simulink model "ad3ab2"  (Simulink 4.00)
settings: Solver=ode45  SolverMode=SingleTasking  StartTime=0.0  StopTime=0.2  RelTol=1e-4  AbsTol=1e-8
CloseFcn:
  | ;slview('closediagram',bdroot);
settings Model: LimitDataPoints=off  BlockReductionOpt=off

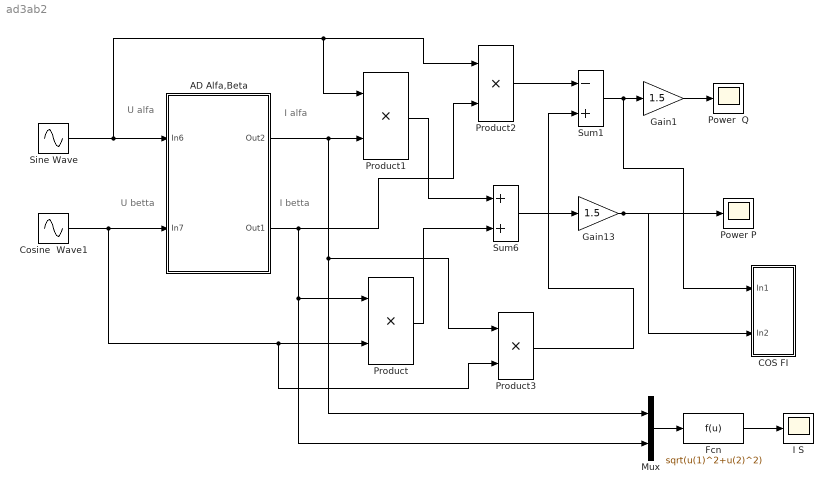
== system ad3ab2 ==
  note: I alfa
  note: I betta
  note: U alfa
  note: U betta
  AD Alfa,Beta : Subsystem
      settings: RTWFcnNameOpts=Auto  RTWFileNameOpts=Auto
  COS FI : Subsystem
      settings: RTWFcnNameOpts=Auto  RTWFileNameOpts=Auto
  Cosine  Wave1 : Sin  SineType=Time-based  Amplitude=311  Bias=0  Frequency=314  Phase=-pi/2  Samples=10  SampleTime=0  Offset=0
  Fcn : Fcn  Expr=sqrt(u(1)^2+u(2)^2)
  Gain1 : Gain  Gain=1.5  Multiplication=Element-wise(K.*u)  SaturateOnIntegerOverflow=on
  Gain13 : Gain  Gain=1.5  Multiplication=Element-wise(K.*u)  SaturateOnIntegerOverflow=on
  I S : Scope
      settings: TickLabels=on  TimeRange=80  YMin=-1  YMax=2  SaveToWorkspace=off  SaveName=ScopeData5  DataFormat=Array  MaxDataPoints=5000
  Mux : Mux  Inputs=2
  Power  Q : Scope
      settings: TickLabels=on  TimeRange=80  YMin=-1  YMax=2  SaveToWorkspace=off  SaveName=ScopeData3  DataFormat=Array  MaxDataPoints=5000
  Power P : Scope
      settings: TickLabels=on  TimeRange=80  YMin=-1  YMax=2  SaveToWorkspace=off  SaveName=ScopeData2  DataFormat=Array  MaxDataPoints=5000
  Product{,1..3} (4 alike) : Product  Inputs=2  Multiplication=Element-wise(.*)  SaturateOnIntegerOverflow=on
  Sine Wave : Sin  SineType=Time-based  Amplitude=311  Bias=0  Frequency=314  Phase=0  Samples=10  SampleTime=0  Offset=0
  Sum1 : Sum  Inputs=-+  SaturateOnIntegerOverflow=on
  Sum6 : Sum  Inputs=++  SaturateOnIntegerOverflow=on
  wires:
  AD Alfa,Beta/1(Out2) -> Product1/2, Product3/1, Mux/1
  Sine Wave/1 -> AD Alfa,Beta/1(In6), Product1/1, Product2/1
  Cosine  Wave1/1 -> AD Alfa,Beta/2(In7), Product/2, Product3/2
  AD Alfa,Beta/2(Out1) -> Product2/2, Product/1, Mux/2
  Product1/1 -> Sum6/1
  Product/1 -> Sum6/2
  Gain13/1 -> Power P/1, COS FI/2(In2)
  Sum6/1 -> Gain13/1
  Product3/1 -> Sum1/2
  Product2/1 -> Sum1/1
  Sum1/1 -> Gain1/1, COS FI/1(In1)
  Gain1/1 -> Power  Q/1
  Fcn/1 -> I S/1
  Mux/1 -> Fcn/1

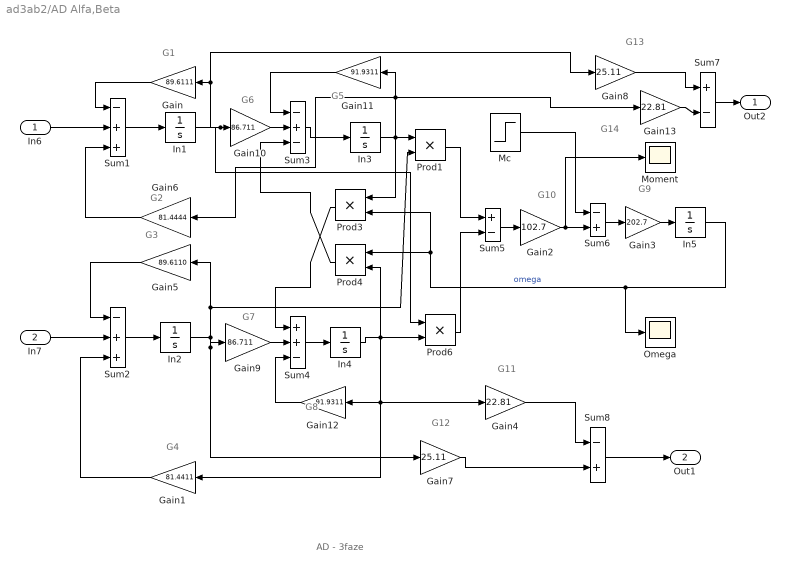
== system ad3ab2/AD Alfa,Beta ==
  note: G1
  note: G2
  note: G3
  note: G4
  note: G10
  note: G9
  note: G6
  note: G7
  note: G8
  note: G5
  note: AD - 3faze
  note: G14
  note: G12
  note: G13
  note: G11
  In6 : Inport  Port=1  LatchInput=off
  In7 : Inport  Port=2  LatchInput=off
  "  Prod1" : Product  Inputs=2  Multiplication=Element-wise(.*)  SaturateOnIntegerOverflow=on
  Gain : Gain  Orientation=left  Gain=89.6111  Multiplication=Element-wise(K.*u)  SaturateOnIntegerOverflow=on
  Gain1 : Gain  Orientation=left  Gain=81.4411  Multiplication=Element-wise(K.*u)  SaturateOnIntegerOverflow=on
  Gain10 : Gain  Gain=86.711  Multiplication=Element-wise(K.*u)  SaturateOnIntegerOverflow=on
  Gain11 : Gain  Orientation=left  Gain=91.9311  Multiplication=Element-wise(K.*u)  SaturateOnIntegerOverflow=on
  Gain12 : Gain  Orientation=left  Gain=91.9311  Multiplication=Element-wise(K.*u)  SaturateOnIntegerOverflow=on
  Gain13 : Gain  Gain=22.81  Multiplication=Element-wise(K.*u)  SaturateOnIntegerOverflow=on
  Gain2 : Gain  Gain=102.7  Multiplication=Element-wise(K.*u)  SaturateOnIntegerOverflow=on
  Gain3 : Gain  Gain=202.7  Multiplication=Element-wise(K.*u)  SaturateOnIntegerOverflow=on
  Gain4 : Gain  Gain=22.81  Multiplication=Element-wise(K.*u)  SaturateOnIntegerOverflow=on
  Gain5 : Gain  Orientation=left  Gain=89.6110  Multiplication=Element-wise(K.*u)  SaturateOnIntegerOverflow=on
  Gain6 : Gain  Orientation=left  Gain=81.4444  Multiplication=Element-wise(K.*u)  SaturateOnIntegerOverflow=on
  Gain7 : Gain  Gain=25.11  Multiplication=Element-wise(K.*u)  SaturateOnIntegerOverflow=on
  Gain8 : Gain  Gain=25.11  Multiplication=Element-wise(K.*u)  SaturateOnIntegerOverflow=on
  Gain9 : Gain  Gain=86.711  Multiplication=Element-wise(K.*u)  SaturateOnIntegerOverflow=on
  In{1..5} (5 alike) : Integrator  ExternalReset=none  InitialConditionSource=internal  InitialCondition=0  LimitOutput=off  UpperSaturationLimit=inf  LowerSaturationLimit=-inf  ShowSaturationPort=off  ShowStatePort=off  AbsoluteTolerance=auto
  Mc : Step  Time=0.1  Before=0.0  After=17.4  SampleTime=0
  Moment : Scope
      settings: TickLabels=on  TimeRange=80  YMin=-1  YMax=2  SaveToWorkspace=off  SaveName=ScopeData  DataFormat=Array  MaxDataPoints=5000
  Omega : Scope
      settings: TickLabels=on  TimeRange=0.2  YMin=-100  YMax=125  SaveToWorkspace=off  DataFormat=Array  MaxDataPoints=5000
  Prod3 : Product  Orientation=left  Inputs=2  Multiplication=Element-wise(.*)  SaturateOnIntegerOverflow=on
  Prod4 : Product  Orientation=left  Inputs=2  Multiplication=Element-wise(.*)  SaturateOnIntegerOverflow=on
  Prod6 : Product  Inputs=2  Multiplication=Element-wise(.*)  SaturateOnIntegerOverflow=on
  Sum1 : Sum  Inputs=-++  SaturateOnIntegerOverflow=on
  Sum2 : Sum  Inputs=-++  SaturateOnIntegerOverflow=on
  Sum3 : Sum  Inputs=-+-  SaturateOnIntegerOverflow=on
  Sum4 : Sum  Inputs=++-  SaturateOnIntegerOverflow=on
  Sum5 : Sum  Inputs=+-  SaturateOnIntegerOverflow=on
  Sum6 : Sum  Inputs=-+  SaturateOnIntegerOverflow=on
  Sum7 : Sum  Inputs=+-  SaturateOnIntegerOverflow=on
  Sum8 : Sum  Inputs=-+  SaturateOnIntegerOverflow=on
  Out2 : Outport  Port=1
  Out1 : Outport  Port=2
  wires:
  Gain/1 -> Sum1/1
  Sum2/1 -> In2/1
  In4/1 -> Prod4/2, Prod6/2, Gain1/1, Gain12/1, Gain4/1
  In3/1 -> Prod3/1, "  Prod1"/1, Gain6/1, Gain11/1, Gain13/1
  Prod6/1 -> Sum5/2
  Sum6/1 -> Gain3/1
  Gain3/1 -> In5/1
  Mc/1 -> Sum6/1
  "  Prod1"/1 -> Sum5/1
  Sum3/1 -> In3/1
  Sum5/1 -> Gain2/1
  Sum1/1 -> In1/1
  In2/1 -> "  Prod1"/2, Gain5/1, Gain9/1, Gain7/1
  In1/1 -> Gain10/1, Gain/1, Gain8/1, Prod6/1
  Gain10/1 -> Sum3/2
  Gain9/1 -> Sum4/2
  Gain5/1 -> Sum2/1
  Prod4/1 -> Sum3/3
  Prod3/1 -> Sum4/1
  Gain2/1 -> Sum6/2, Moment/1
  Gain11/1 -> Sum3/1
  Gain12/1 -> Sum4/3
  In5/1 -> Prod3/2, Prod4/1, Omega/1  "omega"
  Sum4/1 -> In4/1
  Gain7/1 -> Sum8/2
  Gain4/1 -> Sum8/1
  Gain6/1 -> Sum1/3
  Gain1/1 -> Sum2/3
  In7/1 -> Sum2/2
  Gain8/1 -> Sum7/1
  Gain13/1 -> Sum7/2
  In6/1 -> Sum1/2
  Sum8/1 -> Out1/1
  Sum7/1 -> Out2/1

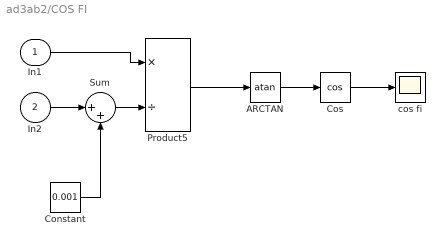
== system ad3ab2/COS FI ==
  In1 : Inport  Port=1  LatchInput=off
  In2 : Inport  Port=2  LatchInput=off
  ARCTAN : Trigonometry  Operator=atan  OutputSignalType=auto
  Constant : Constant  Value=0.001
  Cos : Trigonometry  Operator=cos  OutputSignalType=auto
  Product5 : Product  Inputs=*/  Multiplication=Element-wise(.*)  SaturateOnIntegerOverflow=on
  Sum : Sum  Inputs=|++  SaturateOnIntegerOverflow=on
  cos fi : Scope
      settings: TickLabels=on  TimeRange=0.05  YMin=0  YMax=1  SaveToWorkspace=off  SaveName=ScopeData4  DataFormat=Array  MaxDataPoints=5000
  wires:
  Product5/1 -> ARCTAN/1
  In1/1 -> Product5/1
  Cos/1 -> cos fi/1
  ARCTAN/1 -> Cos/1
  In2/1 -> Sum/1
  Sum/1 -> Product5/2
  Constant/1 -> Sum/2
